simulink model "problem3"  (R2024a)
settings: Solver=VariableStepAuto  StartTime=0.0  StopTime=50  RelTol=1e-3
settings Model: Creator=oxcarxierra  LastModifiedBy=oxcarxierra

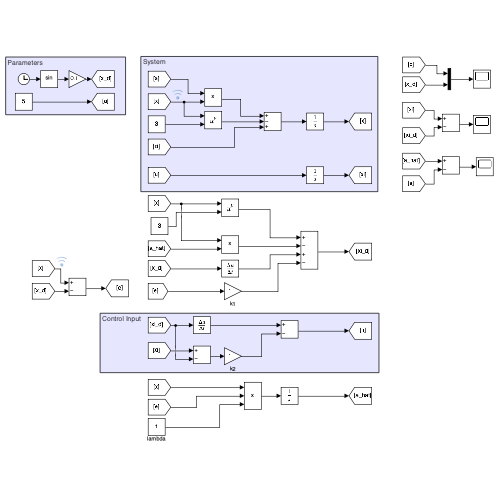
[thumbnail: Simulink's stored preview of the top-level diagram]
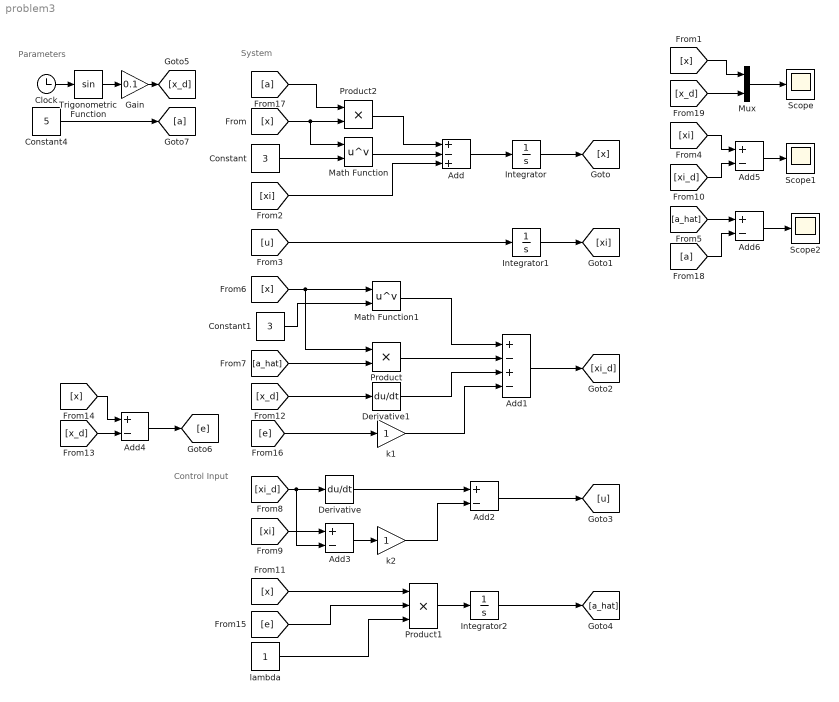
== system problem3 ==
  note: Control Input
  note: Parameters
  note: System
  Add : Sum  Inputs=+-+
  Add1 : Sum  Inputs=+-+-
  Add{2..6} (5 alike) : Sum  Inputs=+-
  Clock : Clock
  Constant : Constant  Value=3
  Constant1 : Constant  Value=3
  Constant4 : Constant  Value=5
  Derivative : Derivative
  Derivative1 : Derivative
  Gain : Gain  Gain=0.1
  Integrator : Integrator
  Integrator1 : Integrator
  Integrator2 : Integrator  InitialCondition=3
  Math Function : Math  Operator=pow
  Math Function1 : Math  Operator=pow
  Mux : Mux  Inputs=2
  Product : Product
  Product1 : Product  Inputs=3
  Product2 : Product
  Scope : Scope
  Scope1 : Scope
  Scope2 : Scope
  Trigonometric Function : Trigonometry
  k1 : Gain
  k2 : Gain
  lambda : Constant
  wires:
  [x] -> Product2/2, Math Function/1
  Product2/1 -> Add/1
  Constant/1 -> Math Function/2
  [xi] -> Add/3
  Math Function/1 -> Add/2
  Add/1 -> Integrator/1
  Integrator/1 -> [x]
  [u] -> Integrator1/1
  Integrator1/1 -> [xi]
  [x] -> Product/1, Math Function1/1
  [a_hat] -> Product/2
  Constant1/1 -> Math Function1/2
  Add1/1 -> [xi_d]
  [xi_d] -> Add3/2, Derivative/1
  Derivative/1 -> Add2/1
  Add2/1 -> [u]
  [xi] -> Add3/1
  Add3/1 -> k2/1
  k2/1 -> Add2/2
  Integrator2/1 -> [a_hat]
  Product1/1 -> Integrator2/1
  [x] -> Product1/1
  [x_d] -> Derivative1/1
  lambda/1 -> Product1/3
  [x] -> Add4/1
  [x_d] -> Add4/2
  Add4/1 -> [e]
  [e] -> Product1/2
  [e] -> k1/1
  Math Function1/1 -> Add1/1
  Product/1 -> Add1/2
  Derivative1/1 -> Add1/3
  k1/1 -> Add1/4
  Add5/1 -> Scope1/1
  [xi] -> Add5/1
  [xi_d] -> Add5/2
  [a_hat] -> Add6/1
  Add6/1 -> Scope2/1
  Constant4/1 -> [a]
  [a] -> Product2/1
  [a] -> Add6/2
  Mux/1 -> Scope/1
  [x] -> Mux/1
  [x_d] -> Mux/2
  Gain/1 -> [x_d]
  Clock/1 -> Trigonometric Function/1
  Trigonometric Function/1 -> Gain/1
